simulink model "kopter_se_zavazim_simulace_2024a"  (R2024a)
settings: Solver=FixedStepAuto  StartTime=0.0  StopTime=5  FixedStep=0.01  RelTol=1e-3
values from neighbouring files (symbols this model uses):
  b_moment = 5.4e-6    (= 5.4e-06)    [parametry_kopter_se_zavazim.m]
  d = 1    [parametry_kopter_se_zavazim.m]
  g = 9.81    [parametry_kopter_se_zavazim.m]
  Ip = m*d^2    (= 1)    [parametry_kopter_se_zavazim.m]
  Ixx = 0.0222    [parametry_kopter_se_zavazim.m]
  Iyy = 0.0222    [parametry_kopter_se_zavazim.m]
  Izz = 0.0429    [parametry_kopter_se_zavazim.m]
  k_thrust = 2.3e-3    (= 0.0023)    [parametry_kopter_se_zavazim.m]
  M = 2    [parametry_kopter_se_zavazim.m]
  m = 1    [parametry_kopter_se_zavazim.m]
  Us_p = [(M+m)*g; 0; 0; 0]    [parametry_kopter_se_zavazim.m]
  Xinit_matrix = [xyz_init; uhly_init; zavazi_init]    [parametry_kopter_se_zavazim.m]
  Xinit_ss = [Xinit_matrix; [0 0 0 0 0 0 0 0]']    [parametry_kopter_se_zavazim.m]
  Xs_p = [0;0;0; 0;0;0; 0;0; 0;0;0; 0;0;0; 0;0]    [parametry_kopter_se_zavazim.m]
undefined symbols (not defined in the file or in its folder): L
libraries: simulink_extras x6
(part 1 of 5)
settings Model: Creator=Admin  LastModifiedBy=Admin

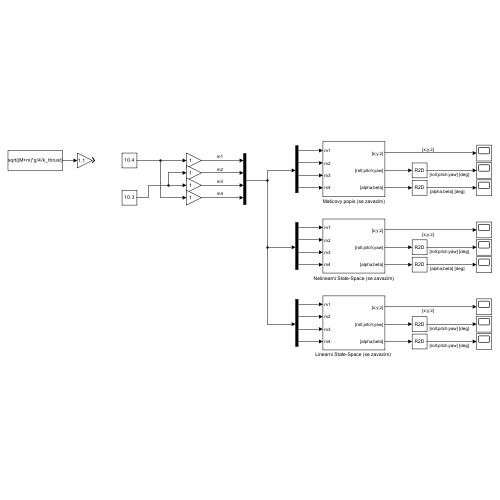
[thumbnail: Simulink's stored preview of the top-level diagram]
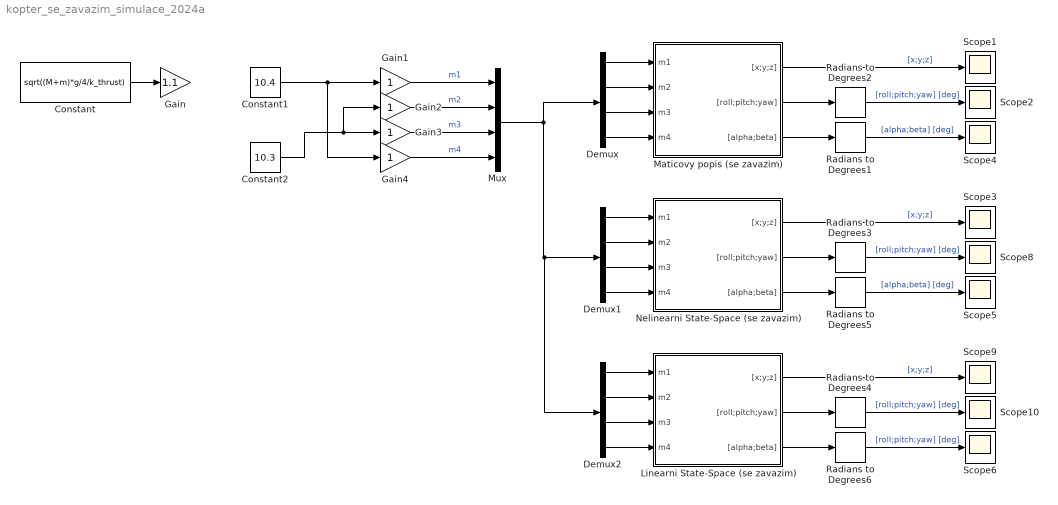
== system kopter_se_zavazim_simulace_2024a ==
  Constant : Constant  Value=sqrt((M+m)*g/4/k_thrust)
  Constant1 : Constant  Value=10.4
  Constant2 : Constant  Value=10.3
  Demux : Demux
  Demux1 : Demux
  Demux2 : Demux
  Gain : Gain  Gain=1.1
  Gain{1..4} (4 alike) : Gain
  "Linearni State-Space (se zavazim) " : Subsystem
  Maticovy popis (se zavazim) : Subsystem
  Mux : Mux
  Nelinearni State-Space (se zavazim) : Subsystem
  Radians to Degrees{1..6} (6 alike) : simulink_extras/Transformations/Radians to Degrees
  Scope{1..6,8..10} (9 alike) : Scope
  wires:
  Gain4/1 -> Mux/4  "m4"
  Constant/1 -> Gain/1
  Gain1/1 -> Mux/1  "m1"
  Gain3/1 -> Mux/3  "m3"
  Gain2/1 -> Mux/2  "m2"
  Maticovy popis (se zavazim)/1("[x;y;z]") -> Scope1/1  "[x;y;z]"
  Radians to Degrees2/1 -> Scope2/1  "[roll;pitch;yaw] [deg]"
  Maticovy popis (se zavazim)/2("[roll;pitch;yaw]") -> Radians to Degrees2/1
  Radians to Degrees3/1 -> Scope8/1  "[roll;pitch;yaw] [deg]"
  Nelinearni State-Space (se zavazim)/1("[x;y;z]") -> Scope3/1  "[x;y;z]"
  Nelinearni State-Space (se zavazim)/2("[roll;pitch;yaw]") -> Radians to Degrees3/1
  Radians to Degrees4/1 -> Scope10/1  "[roll;pitch;yaw] [deg]"
  "Linearni State-Space (se zavazim) "/2("[roll;pitch;yaw]") -> Radians to Degrees4/1
  "Linearni State-Space (se zavazim) "/1("[x;y;z]") -> Scope9/1  "[x;y;z]"
  Constant1/1 -> Gain4/1, Gain1/1
  Maticovy popis (se zavazim)/3("[alpha;beta]") -> Radians to Degrees1/1
  Radians to Degrees1/1 -> Scope4/1  "[alpha;beta] [deg]"
  Demux/1 -> Maticovy popis (se zavazim)/1(m1)
  Demux/2 -> Maticovy popis (se zavazim)/2(m2)
  Demux/3 -> Maticovy popis (se zavazim)/3(m3)
  Demux/4 -> Maticovy popis (se zavazim)/4(m4)
  Mux/1 -> Demux/1, Demux2/1, Demux1/1
  Demux1/1 -> Nelinearni State-Space (se zavazim)/1(m1)
  Demux1/2 -> Nelinearni State-Space (se zavazim)/2(m2)
  Demux1/3 -> Nelinearni State-Space (se zavazim)/3(m3)
  Demux1/4 -> Nelinearni State-Space (se zavazim)/4(m4)
  Radians to Degrees5/1 -> Scope5/1  "[alpha;beta] [deg]"
  Nelinearni State-Space (se zavazim)/3("[alpha;beta]") -> Radians to Degrees5/1
  Demux2/1 -> "Linearni State-Space (se zavazim) "/1(m1)
  Demux2/2 -> "Linearni State-Space (se zavazim) "/2(m2)
  Demux2/3 -> "Linearni State-Space (se zavazim) "/3(m3)
  Demux2/4 -> "Linearni State-Space (se zavazim) "/4(m4)
  Radians to Degrees6/1 -> Scope6/1  "[roll;pitch;yaw] [deg]"
  "Linearni State-Space (se zavazim) "/3("[alpha;beta]") -> Radians to Degrees6/1
  Constant2/1 -> Gain2/1, Gain3/1

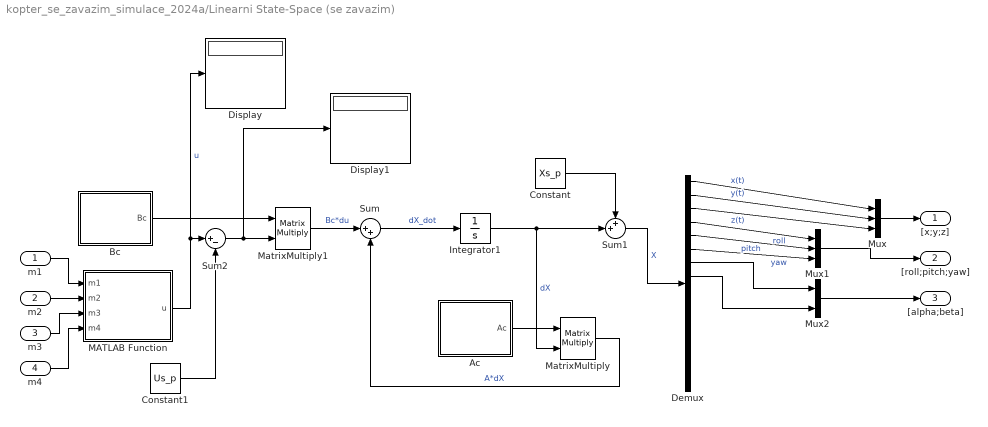
== system kopter_se_zavazim_simulace_2024a/Linearni State-Space (se zavazim)  ==
  m1 : Inport
  m2 : Inport  Port=2
  m3 : Inport  Port=3
  m4 : Inport  Port=4
  Ac : MATLAB Function  TreatAsAtomicUnit=on
  Bc : MATLAB Function  TreatAsAtomicUnit=on
  Constant : Constant  Value=Xs_p
  Constant1 : Constant  Value=Us_p
  Demux : Demux  Outputs=16
  Display : Display
  Display1 : Display
  Integrator1 : Integrator  InitialCondition=Xinit_ss
  MATLAB Function : MATLAB Function  TreatAsAtomicUnit=on
  MatrixMultiply : Product  Multiplication=Matrix(*)
  MatrixMultiply1 : Product  Multiplication=Matrix(*)
  Mux : Mux  Inputs=3
  Mux1 : Mux  Inputs=3
  Mux2 : Mux  Inputs=2
  Sum : Sum  Inputs=|++
  Sum1 : Sum  Inputs=++|
  Sum2 : Sum  Inputs=|+-
  "[x;y;z]" : Outport
  "[roll;pitch;yaw]" : Outport  Port=2
  "[alpha;beta]" : Outport  Port=3
  wires:
  MATLAB Function/1(u) -> Display/1, Sum2/1  "u"
  m3/1 -> MATLAB Function/3(m3)
  m2/1 -> MATLAB Function/2(m2)
  m4/1 -> MATLAB Function/4(m4)
  m1/1 -> MATLAB Function/1(m1)
  Ac/1(Ac) -> MatrixMultiply/1
  Integrator1/1 -> Sum1/2, MatrixMultiply/2  "dX"
  Demux/1 -> Mux/1  "x(t)"
  Demux/2 -> Mux/2  "y(t)"
  Demux/3 -> Mux/3  "z(t)"
  Mux/1 -> "[x;y;z]"/1
  Demux/4 -> Mux1/1  "roll"
  Demux/5 -> Mux1/2  "pitch"
  Demux/6 -> Mux1/3  "yaw"
  Mux1/1 -> "[roll;pitch;yaw]"/1
  Sum/1 -> Integrator1/1  "dX_dot"
  MatrixMultiply1/1 -> Sum/1  "Bc*du"
  MatrixMultiply/1 -> Sum/2  "A*dX"
  Bc/1(Bc) -> MatrixMultiply1/1
  Sum1/1 -> Demux/1  "X"
  Constant/1 -> Sum1/1
  Constant1/1 -> Sum2/2
  Sum2/1 -> Display1/1, MatrixMultiply1/2
  Mux2/1 -> "[alpha;beta]"/1
  Demux/7 -> Mux2/1
  Demux/8 -> Mux2/2

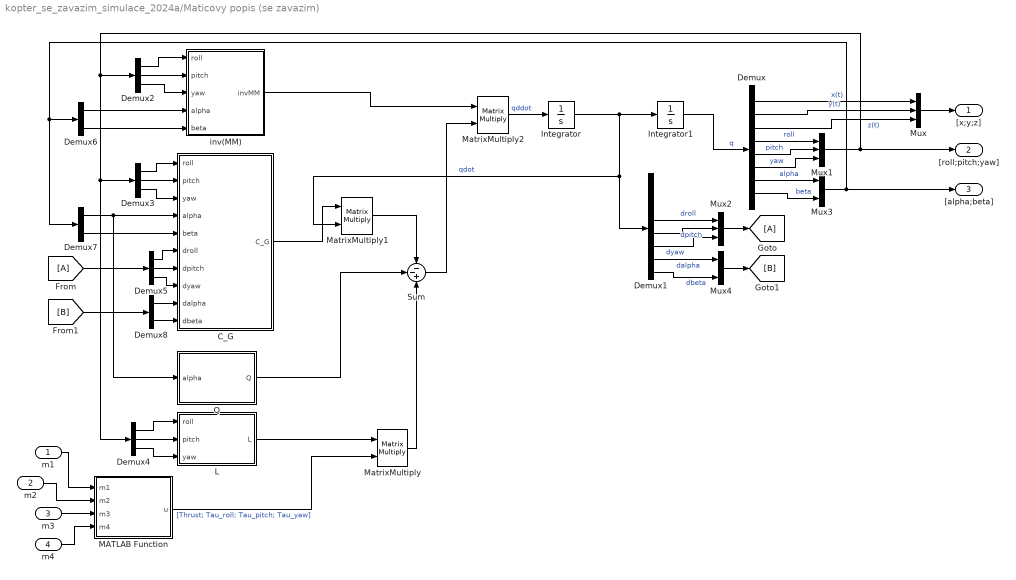
== system kopter_se_zavazim_simulace_2024a/Maticovy popis (se zavazim) ==
  m1 : Inport
  m2 : Inport  Port=2
  m3 : Inport  Port=3
  m4 : Inport  Port=4
  C_G : MATLAB Function  TreatAsAtomicUnit=on
  Demux : Demux  Outputs=8
  Demux1 : Demux  Outputs=8
  Demux{2..5} (4 alike) : Demux  Outputs=3
  Demux6 : Demux  Outputs=2
  Demux7 : Demux  Outputs=2
  Demux8 : Demux  Outputs=2
  From : From
  Goto : Goto
  Integrator : Integrator  InitialCondition=[0;0;0;0;0;0;0;0]
  Integrator1 : Integrator  InitialCondition=Xinit_matrix
  L : MATLAB Function  TreatAsAtomicUnit=on
  MATLAB Function : MATLAB Function  TreatAsAtomicUnit=on
  MatrixMultiply : Product  Multiplication=Matrix(*)
  MatrixMultiply1 : Product  Multiplication=Matrix(*)
  MatrixMultiply2 : Product  Multiplication=Matrix(*)
  Mux : Mux  Inputs=3
  Mux1 : Mux  Inputs=3
  Mux2 : Mux  Inputs=3
  Mux3 : Mux  Inputs=2
  Mux4 : Mux  Inputs=2
  Q : MATLAB Function  TreatAsAtomicUnit=on
  Sum : Sum  Inputs=--+
  inv(MM) : MATLAB Function  TreatAsAtomicUnit=on
  "[x;y;z]" : Outport
  "[roll;pitch;yaw]" : Outport  Port=2
  "[alpha;beta]" : Outport  Port=3
  wires:
  inv(MM)/1(invMM) -> MatrixMultiply2/1
  L/1(L) -> MatrixMultiply/1
  MATLAB Function/1(u) -> MatrixMultiply/2  "[Thrust; Tau_roll; Tau_pitch; Tau_yaw]"
  m3/1 -> MATLAB Function/3(m3)
  m2/1 -> MATLAB Function/2(m2)
  m4/1 -> MATLAB Function/4(m4)
  MatrixMultiply/1 -> Sum/3
  m1/1 -> MATLAB Function/1(m1)
  Q/1(Q) -> Sum/2
  C_G/1(C_G) -> MatrixMultiply1/1
  MatrixMultiply1/1 -> Sum/1
  Sum/1 -> MatrixMultiply2/2
  MatrixMultiply2/1 -> Integrator/1  "qddot"
  Integrator/1 -> MatrixMultiply1/2, Demux1/1, Integrator1/1  "qdot"
  Integrator1/1 -> Demux/1  "q"
  Demux/1 -> Mux/1  "x(t)"
  Demux/2 -> Mux/2  "y(t)"
  Demux/3 -> Mux/3  "z(t)"
  Mux/1 -> "[x;y;z]"/1
  Demux/4 -> Mux1/1  "roll"
  Demux/5 -> Mux1/2  "pitch"
  Demux/6 -> Mux1/3  "yaw"
  Mux1/1 -> "[roll;pitch;yaw]"/1, Demux2/1, Demux3/1, Demux4/1
  Demux1/4 -> Mux2/1  "droll"
  Demux1/5 -> Mux2/2  "dpitch"
  Demux1/6 -> Mux2/3  "dyaw"
  Demux2/1 -> inv(MM)/1(roll)
  Demux2/2 -> inv(MM)/2(pitch)
  Demux2/3 -> inv(MM)/3(yaw)
  Demux3/2 -> C_G/2(pitch)
  Demux3/1 -> C_G/1(roll)
  Demux3/3 -> C_G/3(yaw)
  Demux4/2 -> L/2(pitch)
  Demux4/1 -> L/1(roll)
  Demux4/3 -> L/3(yaw)
  Demux5/2 -> C_G/7(dpitch)
  Demux5/1 -> C_G/6(droll)
  Demux5/3 -> C_G/8(dyaw)
  Demux/7 -> Mux3/1  "alpha"
  Demux/8 -> Mux3/2  "beta"
  Mux3/1 -> "[alpha;beta]"/1, Demux7/1, Demux6/1
  Demux6/1 -> inv(MM)/4(alpha)
  Demux6/2 -> inv(MM)/5(beta)
  Demux7/2 -> C_G/5(beta)
  Demux7/1 -> C_G/4(alpha), Q/1(alpha)
  Demux8/1 -> C_G/9(dalpha)
  Demux8/2 -> C_G/10(dbeta)
  Demux1/7 -> Mux4/1  "dalpha"
  Demux1/8 -> Mux4/2  "dbeta"
  Mux2/1 -> Goto/1
  Mux4/1 -> [B]
  From/1 -> Demux5/1
  [B] -> Demux8/1

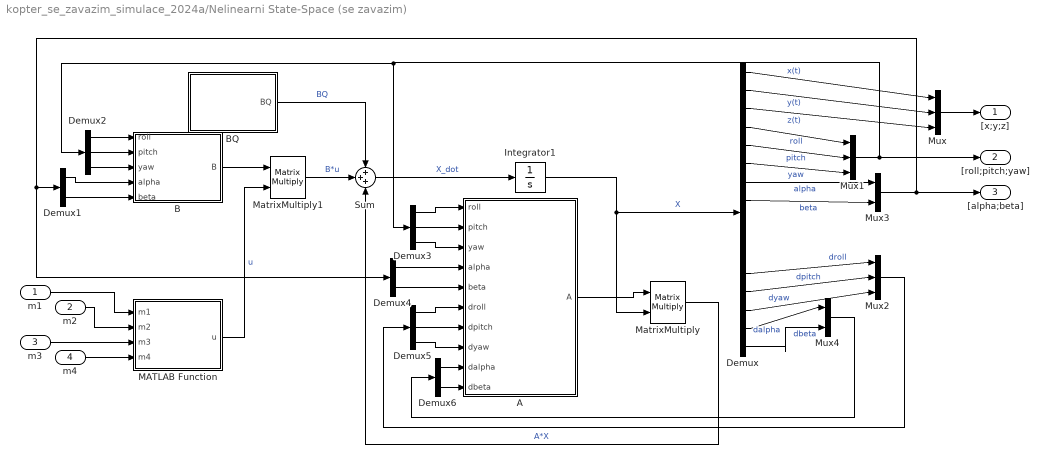
== system kopter_se_zavazim_simulace_2024a/Nelinearni State-Space (se zavazim) ==
  m1 : Inport
  m2 : Inport  Port=2
  m3 : Inport  Port=3
  m4 : Inport  Port=4
  A : MATLAB Function  TreatAsAtomicUnit=on
  B : MATLAB Function  TreatAsAtomicUnit=on
  BQ : MATLAB Function  TreatAsAtomicUnit=on
  Demux : Demux  Outputs=16
  Demux1 : Demux  Outputs=2
  Demux2 : Demux  Outputs=3
  Demux3 : Demux  Outputs=3
  Demux4 : Demux  Outputs=2
  Demux5 : Demux  Outputs=3
  Demux6 : Demux  Outputs=2
  Integrator1 : Integrator  InitialCondition=Xinit_ss
  MATLAB Function : MATLAB Function  TreatAsAtomicUnit=on
  MatrixMultiply : Product  Multiplication=Matrix(*)
  MatrixMultiply1 : Product  Multiplication=Matrix(*)
  Mux : Mux  Inputs=3
  Mux1 : Mux  Inputs=3
  Mux2 : Mux  Inputs=3
  Mux3 : Mux  Inputs=2
  Mux4 : Mux  Inputs=2
  Sum : Sum  Inputs=+++
  "[x;y;z]" : Outport
  "[roll;pitch;yaw]" : Outport  Port=2
  "[alpha;beta]" : Outport  Port=3
  wires:
  MATLAB Function/1(u) -> MatrixMultiply1/2  "u"
  m3/1 -> MATLAB Function/3(m3)
  m2/1 -> MATLAB Function/2(m2)
  m4/1 -> MATLAB Function/4(m4)
  m1/1 -> MATLAB Function/1(m1)
  A/1(A) -> MatrixMultiply/1
  Integrator1/1 -> MatrixMultiply/2, Demux/1  "X"
  Demux/1 -> Mux/1  "x(t)"
  Demux/2 -> Mux/2  "y(t)"
  Demux/3 -> Mux/3  "z(t)"
  Mux/1 -> "[x;y;z]"/1
  Demux/4 -> Mux1/1  "roll"
  Demux/5 -> Mux1/2  "pitch"
  Demux/6 -> Mux1/3  "yaw"
  Mux1/1 -> Demux2/1, Demux3/1, "[roll;pitch;yaw]"/1
  Demux/12 -> Mux2/1  "droll"
  Demux/13 -> Mux2/2  "dpitch"
  Demux/14 -> Mux2/3  "dyaw"
  Demux2/1 -> B/1(roll)
  Demux2/2 -> B/2(pitch)
  Demux2/3 -> B/3(yaw)
  Demux3/2 -> A/2(pitch)
  Demux3/1 -> A/1(roll)
  Demux3/3 -> A/3(yaw)
  Demux5/2 -> A/7(dpitch)
  Demux5/1 -> A/6(droll)
  Demux5/3 -> A/8(dyaw)
  Sum/1 -> Integrator1/1  "X_dot"
  BQ/1(BQ) -> Sum/1  "BQ"
  MatrixMultiply1/1 -> Sum/2  "B*u"
  B/1(B) -> MatrixMultiply1/1
  MatrixMultiply/1 -> Sum/3  "A*X"
  Mux2/1 -> Demux5/1
  Demux/7 -> Mux3/1  "alpha"
  Demux/8 -> Mux3/2  "beta"
  Mux3/1 -> Demux4/1, Demux1/1, "[alpha;beta]"/1
  Demux1/2 -> B/5(beta)
  Demux1/1 -> B/4(alpha)
  Demux4/2 -> A/5(beta)
  Demux4/1 -> A/4(alpha)
  Demux/15 -> Mux4/1  "dalpha"
  Demux/16 -> Mux4/2  "dbeta"
  Demux6/1 -> A/9(dalpha)
  Demux6/2 -> A/10(dbeta)
  Mux4/1 -> Demux6/1

== matlab function kopter_se_zavazim_simulace_2024a/Nelinearni State-Space (se zavazim)/BQ ==
  data: BQ output; g parameter
function BQ = fcn(g)
% Matice vstupu tihy
BQ = [0 0 0 0 0 0 0 0 0 0 -g 0 0 0 0 0]';

== matlab function kopter_se_zavazim_simulace_2024a/Nelinearni State-Space (se zavazim)/MATLAB Function ==
  data: u output; m1 input; m2 input; m3 input; m4 input; k_thrust parameter; b_moment parameter; L parameter
function u = fcn(m1, m2, m3, m4, k_thrust, b_moment, L)

Thrust = k_thrust*(m1^2 + m2^2 + m3^2 + m4^2);
Tau_roll = L*k_thrust*(m1^2 + m4^2 - m2^2 - m3^2);
Tau_pitch = L*k_thrust*(m4^2 + m3^2 - m1^2 - m2^2);
Tau_yaw = b_moment*(m1^2 + m3^2 - m2^2 - m4^2);

u = [Thrust; Tau_roll; Tau_pitch; Tau_yaw];

== matlab function kopter_se_zavazim_simulace_2024a/Linearni State-Space (se zavazim) /Bc ==
  data: M parameter; Bc output; Ixx parameter; Iyy parameter; Izz parameter; m parameter
function Bc = fcn(M, Ixx, Iyy, Izz, m)
% Matice Ac linearizovana

Bc = [
        0,     0,     0,     0;
        0,     0,     0,     0;
        0,     0,     0,     0;
        0,     0,     0,     0;
        0,     0,     0,     0;
        0,     0,     0,     0;
        0,     0,     0,     0;
        0,     0,     0,     0;
        0,     0,     0,     0;
        0,     0,     0,     0;
1/(M + m),     0,     0,     0;
        0, 1/Ixx,     0,     0;
        0,     0, 1/Iyy,     0;
        0,     0,     0, 1/Izz;
        0,     0,     0,     0;
        0,     0,     0,     0];
